simulink model "scan_match"  (R2026a)
settings: Solver=ode1  StopTime=Inf  FixedStep=1/10
PostLoadFcn:
  | qlabs_setup
model workspace (MAT data in the model file):
  lidarStepSize = 0.2
  mainStepSize = Simulink.Parameter
  mainStepSize.Value = Simulink.data.Expression
  mainStepSize.Value.ExpressionString = "qc_get_step_size"
  mainStepSize.Complexity = 'real'
  mainStepSize.Dimensions = -1
  mainStepSize.DataType = 'auto'
  mode = Simulink.Parameter
  mode.Value = 1
  mode.Complexity = 'real'
  mode.Dimensions = [1 1]
  mode.Description = '0 - education speeds via wheel speed commands
    | 1 - education speeds via body speed commands
    | 2 - research speeds via wheel speed commands
    | 3 - research speeds via body speed commands'
  mode.DataType = 'auto'
  realSenseStepSize = Simulink.Parameter
  realSenseStepSize.Value = Simulink.data.Expression
  realSenseStepSize.Value.ExpressionString = "qc_get_step_size*ceil(1/30/qc_get_step_size)"
  realSenseStepSize.Complexity = 'real'
  realSenseStepSize.Dimensions = -1
  realSenseStepSize.DataType = 'auto'
undefined symbols (not defined in the file or in its folder): Point, qc_get_step_size
libraries: quarc_library x14, simulink x1
settings Model: ExtModeTrigDuration=10000  Creator=mbohra  LastModifiedBy=rdu
settings DebuggingCC: UnderspecifiedInitializationDetection=Classic
settings SimscapeCC: SimscapeNominalValues="[{\"value\":\"1\",\"unit\":\"A\"},{\"value\":\"1\",\"unit\":\"bar\"},{\"value\":\"1\",\"unit\":\"cm^2\"},{\"value\":\"1\",\"unit\":\"cm^3/s\"},{\"value\":\"1\",\"unit\":\"kJ/kg\"},{\"value\":\"1\",\"unit\":\"kW\"},{\"value\":\"1\",\"unit\":\"l\"},{\"value\":\"1\",\"unit\":\"N\"},{\"value\":\"1\",\"unit\":\"N*m\"},{\"value\":\"1\",\"unit\":\"V\"}]"  SimscapeLogType=none  SimscapeLogDataHistory=5000.0

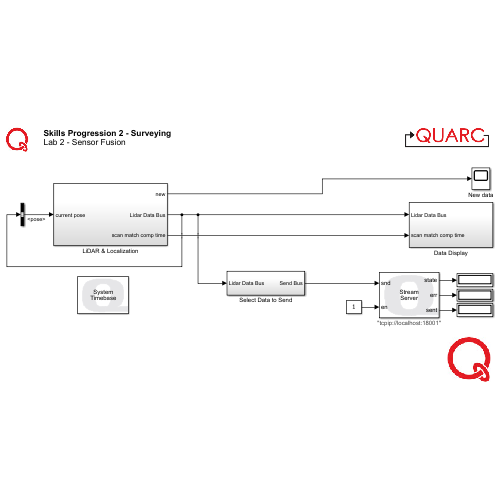
[thumbnail: Simulink's stored preview of the top-level diagram]
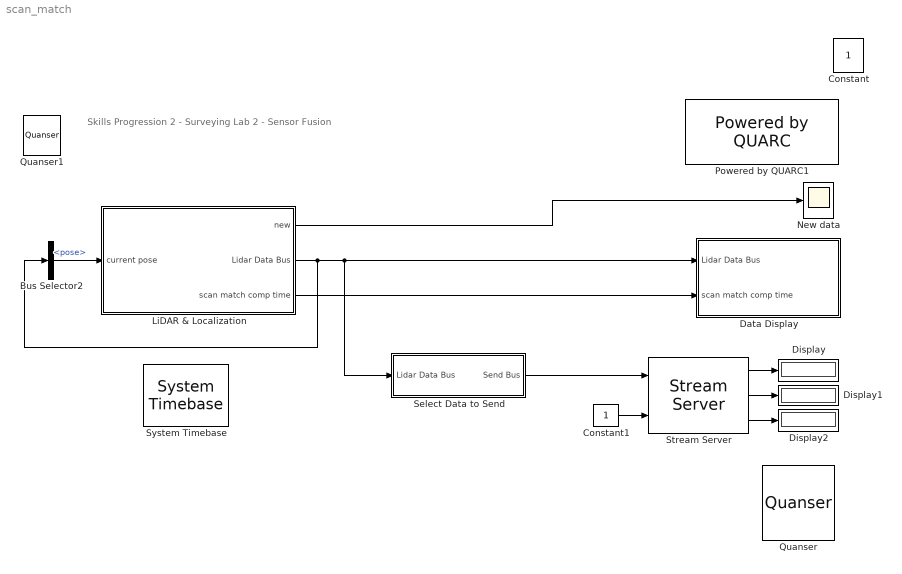
== system scan_match ==
  note: Skills Progression 2 - Surveying
      | Lab 2 - Sensor Fusion
  Bus Selector2 : BusSelector  OutputSignals=pose
  Constant1 : Constant
  Data Display : Subsystem
  Display : Display
  Display1 : Display
  Display2 : Display
  LiDAR & Localization : Subsystem
  New data : Scope
      settings: Title=Hardware Data New?  ActiveDisplayYMinimum=-0.27681268875704879  ActiveDisplayYMaximum=1.0915132332198034  DataLoggingVariableName=ScopeData2
  Powered by QUARC1 : quarc_library/Logos/Powered by QUARC
  Quanser : quarc_library/Logos/Quanser
  Quanser1 : quarc_library/Logos/Quanser
  Select Data to Send : Subsystem
  Stream Server : quarc_library/Communications/Basic/Stream Server  uri_source=Specify via dialog (do not evaluate)  uri=tcpip://localhost:18001  send_buffer_size=(210*2+3)*8*2  receive_buffer_size=3*8*2  byte_order=little endian (Intel - LSB first)  optimization=Minimum latency  send_options=Send most recent data  receive_options=Do not receive data  default_value=[0]  sample_time=qc_get_step_size  active=on  implementation=Use non-blocking I/O  send_fifo_size=2  receive_fifo_size=1000  send_priority=0  receive_priority=0  send_dimensions=off  receive_dimensions=off  max_dimensions=-1  data_type=Inherited via back propagation  type_expr=BusObject
      settings: AttributesFormatString="\"tcpip://localhost:18001\""
  System Timebase : quarc_library/Advanced/Timing/System Timebase  stop_on_overrun=off
      settings: SourceProductName=QUARC Targets
  Constant : Constant  IOType=siggen  VectorParams1D=off  SampleTime=1
  wires:
  LiDAR & Localization/2(Lidar Data Bus) -> Select Data to Send/1(Lidar Data Bus), Data Display/1(Lidar Data Bus), Bus Selector2/1
  Bus Selector2/1 -> LiDAR & Localization/1(current pose)  "<pose>"
  LiDAR & Localization/3(scan match comp time) -> Data Display/2(scan match comp time)
  Stream Server/2 -> Display1/1
  Stream Server/1 -> Display/1
  Constant1/1 -> Stream Server/2
  Stream Server/3 -> Display2/1
  LiDAR & Localization/1(new) -> New data/1
  Select Data to Send/1(Send Bus) -> Stream Server/1

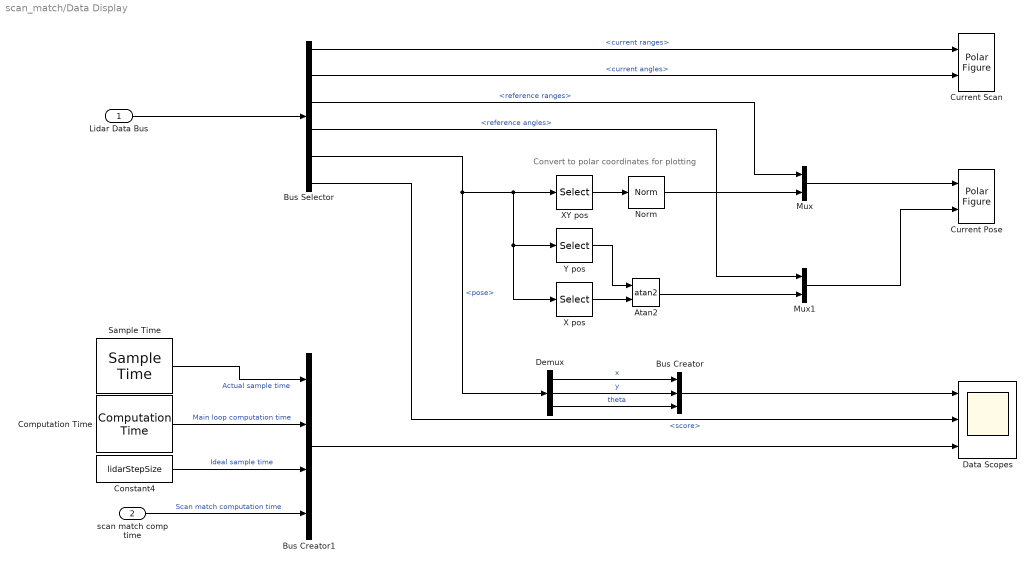
== system scan_match/Data Display ==
  note: Convert to polar coordinates for plotting
  Lidar Data Bus : Inport
  scan match comp time : Inport  Port=2
  Atan2 : Trigonometry  Operator=atan2
  Bus Creator : BusCreator  Inputs=3
  Bus Creator1 : BusCreator  Inputs=4
  Bus Selector : BusSelector  OutputSignals=current ranges,current angles,reference ranges,reference angles,pose,score
  Computation Time : quarc_library/Sources/Time/Computation Time  sample_time=qc_get_step_size  use_model=on  use_cpu_time=off
  Constant4 : Constant  Value=lidarStepSize
  Current Pose : quarc_library/Sinks/Figures/Polar Figure  figure_mode=Use figure window  figure_tag=figure1  axes_tag=axes1  plot_mode=Frame-based  minimum_rho=0  maximum_rho=2  minimum_theta=0  maximum_theta=360  zero_location=right  direction=counterclockwise  buffer_size=2  update_rate=10  sample_time=-1  initial_position="3108   275   471   457"  initial_visibility=off  line1_style=None  line1_width=0.5  line1_color=[1 0 0]  marker1=Point (.)  marker1_size=6  marker1_edge_color=[1 0 0]  marker1_face_color=[1 0 0]  line2_style=Solid line (-)  line2_width=0.5  line2_color=[0.85098 0.32549 0.0980392]  marker2=None  marker2_size=6  marker2_edge_color=[0.85098 0.32549 0.0980392]  marker2_face_color=[0.85098 0.32549 0.0980392]  line3_style=Solid line (-)  line3_width=0.5  line3_color=[0.929412 0.694118 0.12549]  marker3=None  marker3_size=6  marker3_edge_color=[0.929412 0.694118 0.12549]  marker3_face_color=[0.929412 0.694118 0.12549]  line4_style=Solid line (-)  line4_width=0.5  line4_color=[0.494118 0.184314 0.556863]  marker4=None  marker4_size=6  marker4_edge_color=[0.494118 0.184314 0.556863]  marker4_face_color=[0.494118 0.184314 0.556863]  line5_style=Solid line (-)  line5_width=0.5  line5_color=[0.466667 0.67451 0.188235]  marker5=None  marker5_size=6  marker5_edge_color=[0.466667 0.67451 0.188235]  marker5_face_color=[0.466667 0.67451 0.188235]
      settings: SourceProductName=QUARC Targets
  Current Scan : quarc_library/Sinks/Figures/Polar Figure  figure_mode=Use figure window  figure_tag=figure1  axes_tag=axes1  plot_mode=Time-based  minimum_rho=0  maximum_rho=4  minimum_theta=0  maximum_theta=360  zero_location=right  direction=counterclockwise  buffer_size=2  update_rate=1  sample_time=-1  initial_position="112  209  940  693"  initial_visibility=off  line1_style=None  line1_width=0.5  line1_color=[1 0 0]  marker1=Point (.)  marker1_size=6  marker1_edge_color=[1 0 0]  marker1_face_color=[1 0 0]  line2_style=Solid line (-)  line2_width=0.5  line2_color=[0.85098 0.32549 0.0980392]  marker2=None  marker2_size=6  marker2_edge_color=[0.85098 0.32549 0.0980392]  marker2_face_color=[0.85098 0.32549 0.0980392]  line3_style=Solid line (-)  line3_width=0.5  line3_color=[0.929412 0.694118 0.12549]  marker3=None  marker3_size=6  marker3_edge_color=[0.929412 0.694118 0.12549]  marker3_face_color=[0.929412 0.694118 0.12549]  line4_style=Solid line (-)  line4_width=0.5  line4_color=[0.494118 0.184314 0.556863]  marker4=None  marker4_size=6  marker4_edge_color=[0.494118 0.184314 0.556863]  marker4_face_color=[0.494118 0.184314 0.556863]  line5_style=Solid line (-)  line5_width=0.5  line5_color=[0.466667 0.67451 0.188235]  marker5=None  marker5_size=6  marker5_edge_color=[0.466667 0.67451 0.188235]  marker5_face_color=[0.466667 0.67451 0.188235]
      settings: SourceProductName=QUARC Targets
  Data Scopes : Scope  NumInputPorts=3
      settings: ActiveDisplayString=3  Title=Timing  ActiveDisplayYMinimum=-0.034864181774455522  ActiveDisplayYMaximum=0.138720971183178
  Demux : Demux  Outputs=3
  Mux : Mux  Inputs=2
  Mux1 : Mux  Inputs=2
  Norm : quarc_library/Math Operations/Vectors/Norm
      settings: SourceProductName=QUARC Targets
  Sample Time : quarc_library/Sources/Time/Sample Time  Priority=-99  sample_time=qc_get_step_size
  X pos : Selector  InputPortWidth=3  IndexOptions=Index vector (dialog)  Indices=[1]  OutputSizes=1
  "XY pos " : Selector  InputPortWidth=3  IndexOptions=Index vector (dialog)  Indices=[1 2]  OutputSizes=1
  Y pos : Selector  InputPortWidth=3  IndexOptions=Index vector (dialog)  Indices=2  OutputSizes=1
  wires:
  Demux/3 -> Bus Creator/3  "theta"
  Demux/2 -> Bus Creator/2  "y"
  Demux/1 -> Bus Creator/1  "x"
  Bus Creator/1 -> Data Scopes/1
  Bus Selector/6 -> Data Scopes/2  "<score>"
  Sample Time/1 -> Bus Creator1/1  "Actual sample time"
  Computation Time/1 -> Bus Creator1/2  "Main loop computation time"
  Constant4/1 -> Bus Creator1/3  "Ideal sample time"
  Bus Creator1/1 -> Data Scopes/3
  scan match comp time/1 -> Bus Creator1/4  "Scan match computation time"
  Bus Selector/2 -> Current Scan/2  "<current angles>"
  Y pos/1 -> Atan2/1
  Bus Selector/3 -> Mux/1  "<reference ranges>"
  Bus Selector/4 -> Mux1/1  "<reference angles>"
  Bus Selector/1 -> Current Scan/1  "<current ranges>"
  Atan2/1 -> Mux1/2
  Bus Selector/5 -> Demux/1, X pos/1, Y pos/1, "XY pos "/1  "<pose>"
  Norm/1 -> Mux/2
  X pos/1 -> Atan2/2
  "XY pos "/1 -> Norm/1
  Lidar Data Bus/1 -> Bus Selector/1
  Mux/1 -> Current Pose/1
  Mux1/1 -> Current Pose/2

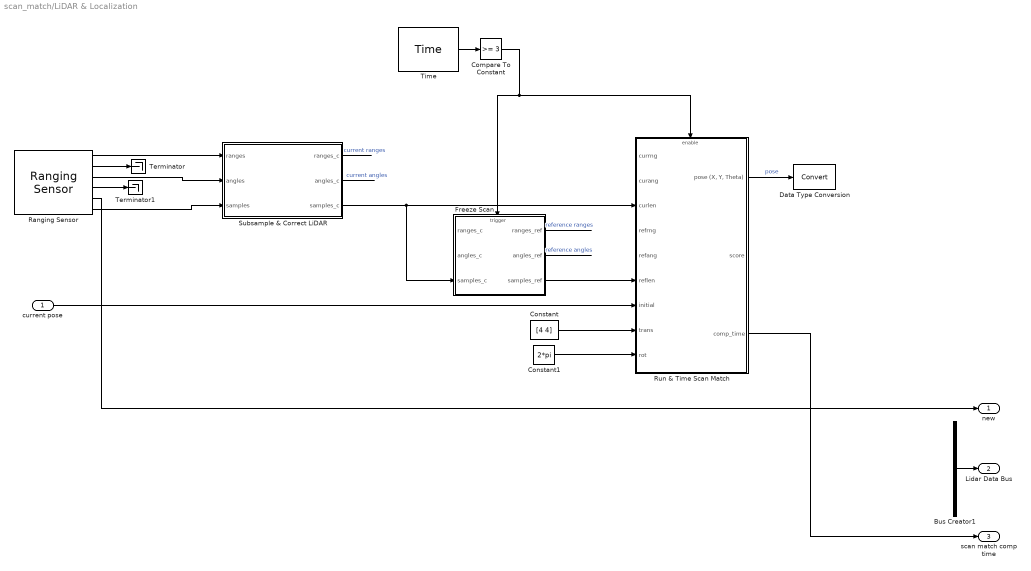
== system scan_match/LiDAR & Localization ==
  current pose : Inport
  Bus Creator1 : BusCreator  Inputs=6
  Compare To Constant : simulink/Logic and Bit Operations/Compare To Constant  relop=>=  const=3  OutDataTypeStr=boolean
  Constant : Constant  Value=[4 4]
  Constant1 : Constant  Value=2*pi
  Data Type Conversion : DataTypeConversion  SaturateOnIntegerOverflow=off  RndMeth=Floor
  Freeze Scan : Subsystem  TreatAsAtomicUnit=on
  Ranging Sensor : quarc_library/Devices/Third-Party/Sensors/Ranging Sensor  sensor_type=Leishen M10P LIDAR  uri=tcpip://localhost:18918  ranging_distance=Short  timing_budget=0.033  measurement_period=0.0005  output_mode=Fixed-size output  samples_per_revolution=1680  max_distance=0.050  max_angle=5  sample_time=qc_get_step_size  show_versions=off  active=on
      settings: SourceProductName=QUARC Targets
  "Run & Time Scan Match " : Subsystem
  Subsample & Correct LiDAR : Subsystem
  Terminator : Terminator
  Terminator1 : Terminator
  Time : quarc_library/Sources/Time/Time  time_source=Wall clock  sample_time=mainStepSize
  new : Outport
  Lidar Data Bus : Outport  Port=2
  scan match comp time : Outport  Port=3
  wires:
  Ranging Sensor/5 -> new/1
  Ranging Sensor/2 -> Terminator/1
  Ranging Sensor/4 -> Terminator1/1
  Compare To Constant/1 -> "Run & Time Scan Match "/Enable, Freeze Scan/Trigger
  "Run & Time Scan Match "/1("pose (X, Y, Theta)") -> Data Type Conversion/1  "pose"
  Freeze Scan/3(samples_ref) -> "Run & Time Scan Match "/6(reflen)
  Subsample & Correct LiDAR/3(samples_c) -> Freeze Scan/3(samples_c), "Run & Time Scan Match "/3(curlen)
  Time/1 -> Compare To Constant/1
  Bus Creator1/1 -> Lidar Data Bus/1
  current pose/1 -> "Run & Time Scan Match "/7(initial)
  Constant/1 -> "Run & Time Scan Match "/8(trans)
  Constant1/1 -> "Run & Time Scan Match "/9(rot)
  "Run & Time Scan Match "/3(comp_time) -> scan match comp time/1
  Ranging Sensor/1 -> Subsample & Correct LiDAR/1(ranges)
  Ranging Sensor/3 -> Subsample & Correct LiDAR/2(angles)
  Ranging Sensor/6 -> Subsample & Correct LiDAR/3(samples)
  ? -> Freeze Scan/2(angles_c)
  ? -> Freeze Scan/1(ranges_c)
  Subsample & Correct LiDAR/2(angles_c) -> ?  "current angles"
  Subsample & Correct LiDAR/1(ranges_c) -> ?  "current ranges"
  Freeze Scan/1(ranges_ref) -> ?  "reference ranges"
  Freeze Scan/2(angles_ref) -> ?  "reference angles"
  ? -> Bus Creator1/1  "current ranges"
  ? -> Bus Creator1/2  "current angles"
  ? -> Bus Creator1/3  "reference ranges"
  ? -> Bus Creator1/4  "reference angles"
  ? -> Bus Creator1/5  "pose"
  ? -> Bus Creator1/6  "score"

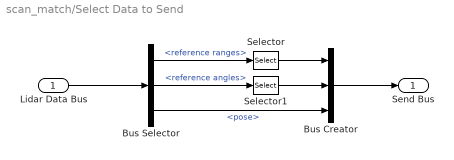
== system scan_match/Select Data to Send ==
  Lidar Data Bus : Inport
  Bus Creator : BusCreator  Inputs=3
  Bus Selector : BusSelector  OutputSignals=reference ranges,reference angles,pose
  Selector : Selector  InputPortWidth=420  IndexOptions=Index vector (dialog)  Indices=[1:2:420]  OutputSizes=1
  Selector1 : Selector  InputPortWidth=420  IndexOptions=Index vector (dialog)  Indices=[1:2:420]  OutputSizes=1
  Send Bus : Outport
  wires:
  Bus Selector/1 -> Selector/1  "<reference ranges>"
  Bus Creator/1 -> Send Bus/1
  Bus Selector/3 -> Bus Creator/3  "<pose>"
  Selector1/1 -> Bus Creator/2
  Selector/1 -> Bus Creator/1
  Lidar Data Bus/1 -> Bus Selector/1
  Bus Selector/2 -> Selector1/1  "<reference angles>"

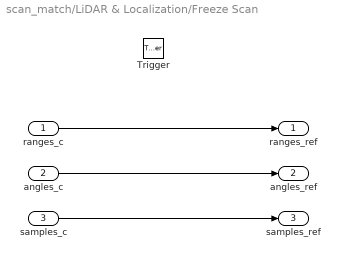
== system scan_match/LiDAR & Localization/Freeze Scan ==
  ranges_c : Inport
  angles_c : Inport  Port=2
  samples_c : Inport  Port=3
  Trigger : TriggerPort  VariantControl=(inherit)  InitialTriggerSignalState=zero
  ranges_ref : Outport
  angles_ref : Outport  Port=2
  samples_ref : Outport  Port=3
  wires:
  ranges_c/1 -> ranges_ref/1
  angles_c/1 -> angles_ref/1
  samples_c/1 -> samples_ref/1

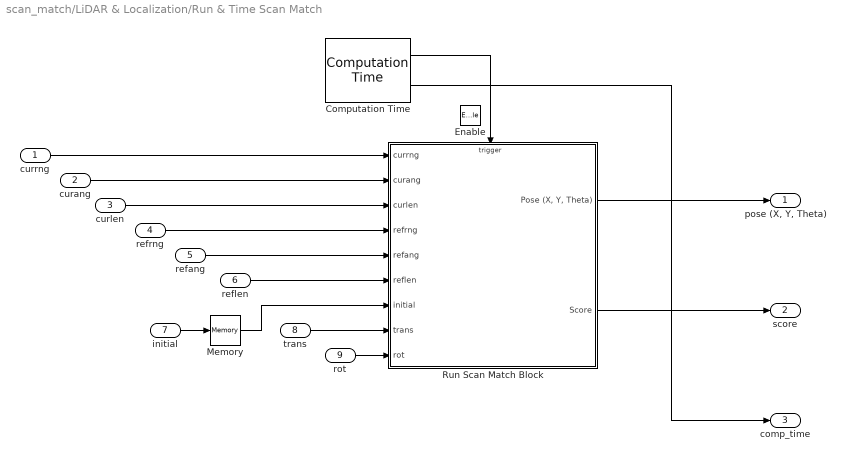
== system scan_match/LiDAR & Localization/Run & Time Scan Match  ==
  currng : Inport
  curang : Inport  Port=2
  curlen : Inport  Port=3
  refrng : Inport  Port=4
  refang : Inport  Port=5
  reflen : Inport  Port=6
  initial : Inport  Port=7
  trans : Inport  Port=8
  rot : Inport  Port=9
  Enable : EnablePort
  Computation Time : quarc_library/Sources/Time/Computation Time  sample_time=qc_get_step_size  use_model=off  use_cpu_time=off
  Memory : Memory  InheritSampleTime=on
  "Run Scan Match Block " : Subsystem  TreatAsAtomicUnit=on
  "pose (X, Y, Theta)" : Outport
  score : Outport  Port=2
  comp_time : Outport  Port=3
  wires:
  currng/1 -> "Run Scan Match Block "/1(currng)
  curang/1 -> "Run Scan Match Block "/2(curang)
  curlen/1 -> "Run Scan Match Block "/3(curlen)
  refrng/1 -> "Run Scan Match Block "/4(refrng)
  refang/1 -> "Run Scan Match Block "/5(refang)
  reflen/1 -> "Run Scan Match Block "/6(reflen)
  initial/1 -> Memory/1
  trans/1 -> "Run Scan Match Block "/8(trans)
  rot/1 -> "Run Scan Match Block "/9(rot)
  Computation Time/1 -> "Run Scan Match Block "/Trigger
  Computation Time/2 -> comp_time/1
  "Run Scan Match Block "/1("Pose (X, Y, Theta)") -> "pose (X, Y, Theta)"/1
  "Run Scan Match Block "/2(Score) -> score/1
  Memory/1 -> "Run Scan Match Block "/7(initial)

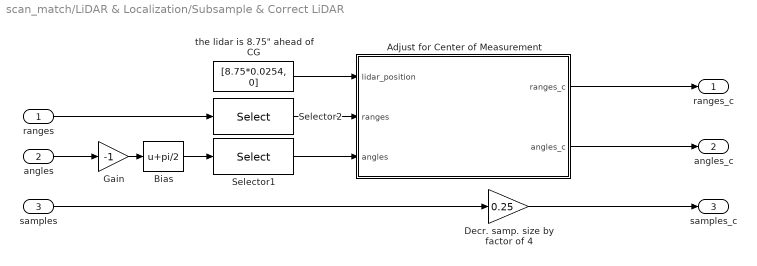
== system scan_match/LiDAR & Localization/Subsample & Correct LiDAR ==
  ranges : Inport
  angles : Inport  Port=2
  samples : Inport  Port=3
  Adjust for Center of Measurement : MATLAB Function  TreatAsAtomicUnit=on
  Bias : Bias  Bias=pi/2  SaturateOnIntegerOverflow=off
  "Decr. samp. size by factor of 4 " : Gain  Gain=0.25  OutDataTypeStr=int32
  Gain : Gain  Gain=-1
  Selector1 : Selector  InputPortWidth=1680  IndexOptions=Index vector (dialog)  Indices=[1:4:1677]  OutputSizes=1
  Selector2 : Selector  InputPortWidth=1680  IndexOptions=Index vector (dialog)  Indices=[1:4:1677]  OutputSizes=1
  "the lidar is 8.75\" ahead of CG" : Constant  Value=[8.75*0.0254, 0]  SampleTime=lidarStepSize
  ranges_c : Outport
  angles_c : Outport  Port=2
  samples_c : Outport  Port=3
  wires:
  "the lidar is 8.75\" ahead of CG"/1 -> Adjust for Center of Measurement/1(lidar_position)
  Selector2/1 -> Adjust for Center of Measurement/2(ranges)
  angles/1 -> Gain/1
  Bias/1 -> Selector1/1
  samples/1 -> "Decr. samp. size by factor of 4 "/1
  Gain/1 -> Bias/1
  ranges/1 -> Selector2/1
  Selector1/1 -> Adjust for Center of Measurement/3(angles)
  Adjust for Center of Measurement/1(ranges_c) -> ranges_c/1
  Adjust for Center of Measurement/2(angles_c) -> angles_c/1
  "Decr. samp. size by factor of 4 "/1 -> samples_c/1

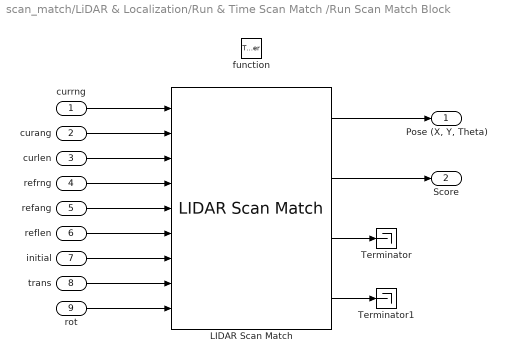
== system scan_match/LiDAR & Localization/Run & Time Scan Match /Run Scan Match Block  ==
  currng : Inport
  curang : Inport  Port=2
  curlen : Inport  Port=3
  refrng : Inport  Port=4
  refang : Inport  Port=5
  reflen : Inport  Port=6
  initial : Inport  Port=7
  trans : Inport  Port=8
  rot : Inport  Port=9
  function : TriggerPort  TriggerType=function-call  VariantControl=(inherit)  SampleTimeType=periodic  SampleTime=qc_get_step_size
  LIDAR Scan Match : quarc_library/Image Processing/Generic/LIDAR Scan Match  mode=Fixed input with size  resolution=10  max_range=5  use_initial_pose=on
      settings: SourceProductName=QUARC Targets
  Terminator : Terminator
  Terminator1 : Terminator
  "Pose (X, Y, Theta)" : Outport
  Score : Outport  Port=2
  wires:
  rot/1 -> LIDAR Scan Match/9
  LIDAR Scan Match/2 -> Score/1
  trans/1 -> LIDAR Scan Match/8
  initial/1 -> LIDAR Scan Match/7
  refang/1 -> LIDAR Scan Match/5
  reflen/1 -> LIDAR Scan Match/6
  LIDAR Scan Match/4 -> Terminator1/1
  currng/1 -> LIDAR Scan Match/1
  LIDAR Scan Match/1 -> "Pose (X, Y, Theta)"/1
  curang/1 -> LIDAR Scan Match/2
  LIDAR Scan Match/3 -> Terminator/1
  curlen/1 -> LIDAR Scan Match/3
  refrng/1 -> LIDAR Scan Match/4

== matlab function scan_match/LiDAR & Localization/Subsample & Correct LiDAR/Adjust for Center of Measurement ==
  data: lidar_position input; ranges input; ranges_c output; angles input; angles_c output
function [ranges_c,angles_c] = correct_lidar(lidar_position, ranges,angles)

% Convert lidar data from polar into cartesian, and add lidar position
% Then convert back into polar coordinates
%-------Replace the following line with your code---------%
ranges_c = ranges;
angles_c = angles./angles;
%---------------------------------------------------------%

end
